simulink model "linear_Einspurmodel"  (R2025b)
settings: Solver=ode4  StartTime=0.0  StopTime=400  FixedStep=5e-05  RelTol=1e-8
values from neighbouring files (symbols this model uses):
  v = 18    [Aufgabe4.m]
settings Model: Creator=jonas  LastModifiedBy=fisch
settings DataIOCC: ExternalInput=u_ext  LoadExternalInput=on

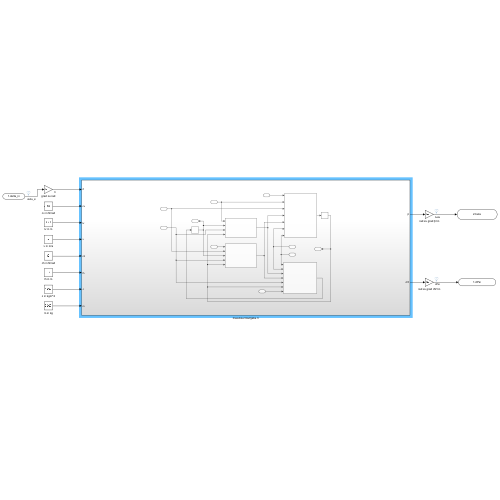
[thumbnail: Simulink's stored preview of the top-level diagram]
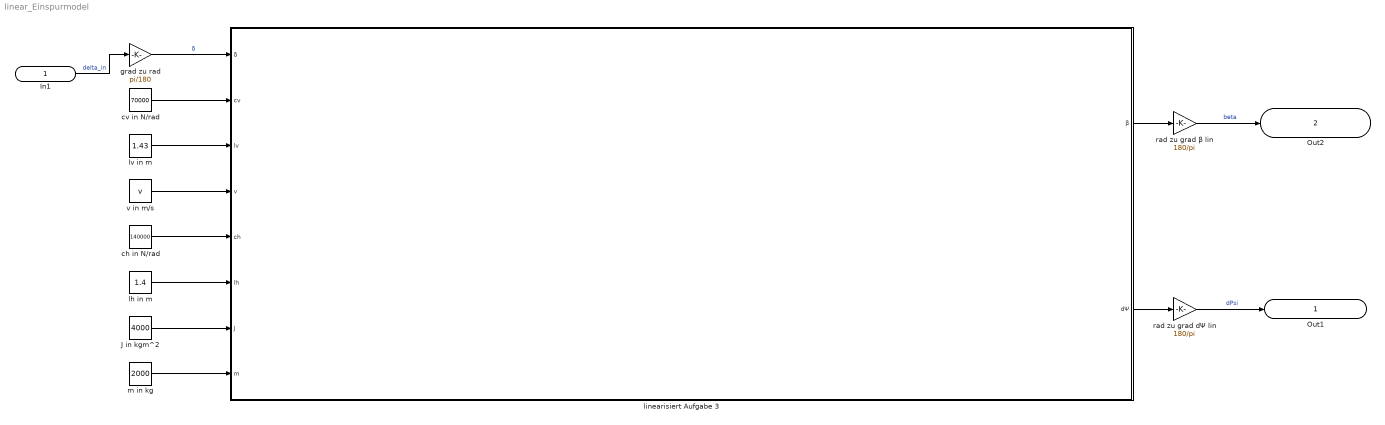
== system linear_Einspurmodel ==
  In1 : Inport
  J in kgm^2 : Constant  Value=4000
  ch in N/rad : Constant  Value=140000
  cv in N/rad : Constant  Value=70000
  grad zu rad : Gain  Gain=pi/180
  lh in m : Constant  Value=1.4
  linearisiert Aufgabe 3 : Subsystem
  lv in m : Constant  Value=1.43
  m in kg : Constant  Value=2000
  rad zu grad dΨ lin : Gain  Gain=180/pi
  rad zu grad β lin : Gain  Gain=180/pi
  v in m/s : Constant  Value=v
  Out1 : Outport
  Out2 : Outport  Port=2
  wires:
  In1/1 -> grad zu rad/1  "delta_in"
  grad zu rad/1 -> linearisiert Aufgabe 3/1(δ)  "δ"
  cv in N/rad/1 -> linearisiert Aufgabe 3/2(cv)
  lv in m/1 -> linearisiert Aufgabe 3/3(lv)
  v in m/s/1 -> linearisiert Aufgabe 3/4(v)
  ch in N/rad/1 -> linearisiert Aufgabe 3/5(ch)
  lh in m/1 -> linearisiert Aufgabe 3/6(lh)
  J in kgm^2/1 -> linearisiert Aufgabe 3/7(J)
  m in kg/1 -> linearisiert Aufgabe 3/8(m)
  linearisiert Aufgabe 3/1(β) -> rad zu grad β lin/1
  linearisiert Aufgabe 3/2(dΨ) -> rad zu grad dΨ lin/1
  rad zu grad dΨ lin/1 -> Out1/1  "dPsi"
  rad zu grad β lin/1 -> Out2/1  "beta"

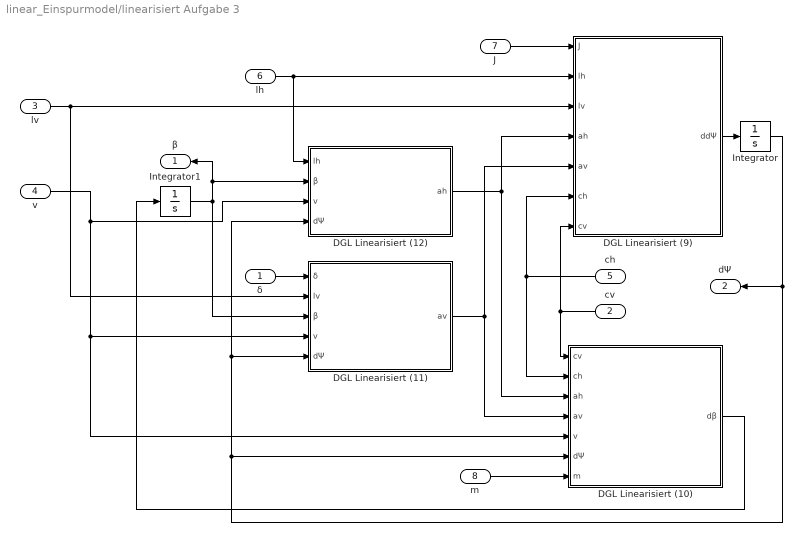
== system linear_Einspurmodel/linearisiert Aufgabe 3 ==
  δ : Inport
  cv : Inport  Port=2
  lv : Inport  Port=3
  v : Inport  Port=4
  ch : Inport  Port=5
  lh : Inport  Port=6
  J : Inport  Port=7
  m : Inport  Port=8
  DGL Linearisiert (10) : Subsystem
  DGL Linearisiert (11) : Subsystem
  DGL Linearisiert (12) : Subsystem
  DGL Linearisiert (9) : Subsystem
  Integrator : Integrator
  Integrator1 : Integrator
  β : Outport
  dΨ : Outport  Port=2
  wires:
  DGL Linearisiert (10)/1(dβ) -> Integrator1/1
  DGL Linearisiert (12)/1(ah) -> DGL Linearisiert (10)/3(ah), DGL Linearisiert (9)/4(ah)
  ch/1 -> DGL Linearisiert (9)/6(ch), DGL Linearisiert (10)/2(ch)
  Integrator/1 -> DGL Linearisiert (10)/6(dΨ), DGL Linearisiert (11)/5(dΨ), DGL Linearisiert (12)/4(dΨ), dΨ/1
  DGL Linearisiert (9)/1(ddΨ) -> Integrator/1
  Integrator1/1 -> DGL Linearisiert (12)/2(β), β/1, DGL Linearisiert (11)/3(β)
  δ/1 -> DGL Linearisiert (11)/1(δ)
  lh/1 -> DGL Linearisiert (12)/1(lh), DGL Linearisiert (9)/2(lh)
  DGL Linearisiert (11)/1(av) -> DGL Linearisiert (10)/4(av), DGL Linearisiert (9)/5(av)
  lv/1 -> DGL Linearisiert (11)/2(lv), DGL Linearisiert (9)/3(lv)
  cv/1 -> DGL Linearisiert (9)/7(cv), DGL Linearisiert (10)/1(cv)
  J/1 -> DGL Linearisiert (9)/1(J)
  v/1 -> DGL Linearisiert (10)/5(v), DGL Linearisiert (11)/4(v), DGL Linearisiert (12)/3(v)
  m/1 -> DGL Linearisiert (10)/7(m)

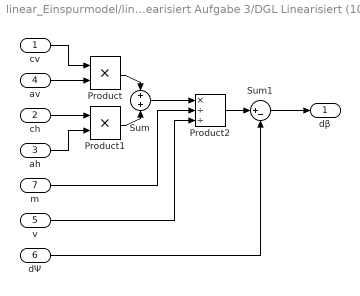
== system linear_Einspurmodel/linearisiert Aufgabe 3/DGL Linearisiert (10) ==
  cv : Inport
  ch : Inport  Port=2
  ah : Inport  Port=3
  av : Inport  Port=4
  v : Inport  Port=5
  dΨ : Inport  Port=6
  m : Inport  Port=7
  Product : Product  Inputs=**
  Product1 : Product  Inputs=**
  Product2 : Product  Inputs=*//
  Sum : Sum  Inputs=+|+
  Sum1 : Sum  Inputs=|+-
  dβ : Outport
  wires:
  Product/1 -> Sum/1
  m/1 -> Product2/2
  cv/1 -> Product/1
  Product2/1 -> Sum1/1
  Product1/1 -> Sum/2
  Sum/1 -> Product2/1
  Sum1/1 -> dβ/1
  av/1 -> Product/2
  v/1 -> Product2/3
  dΨ/1 -> Sum1/2
  ah/1 -> Product1/2
  ch/1 -> Product1/1

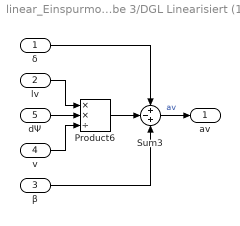
== system linear_Einspurmodel/linearisiert Aufgabe 3/DGL Linearisiert (11) ==
  δ : Inport
  lv : Inport  Port=2
  β : Inport  Port=3
  v : Inport  Port=4
  dΨ : Inport  Port=5
  Product6 : Product  Inputs=**/
  Sum3 : Sum  Inputs=+-+
  av : Outport
  wires:
  lv/1 -> Product6/1
  β/1 -> Sum3/3
  Product6/1 -> Sum3/2
  dΨ/1 -> Product6/2
  Sum3/1 -> av/1  "av"
  v/1 -> Product6/3
  δ/1 -> Sum3/1

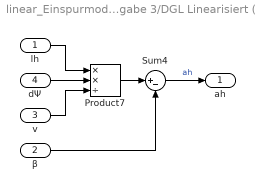
== system linear_Einspurmodel/linearisiert Aufgabe 3/DGL Linearisiert (12) ==
  lh : Inport
  β : Inport  Port=2
  v : Inport  Port=3
  dΨ : Inport  Port=4
  Product7 : Product  Inputs=**/
  Sum4 : Sum  Inputs=|+-
  ah : Outport
  wires:
  Product7/1 -> Sum4/1
  dΨ/1 -> Product7/2
  β/1 -> Sum4/2
  lh/1 -> Product7/1
  v/1 -> Product7/3
  Sum4/1 -> ah/1  "ah"

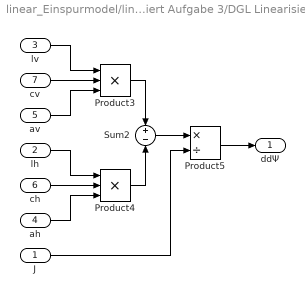
== system linear_Einspurmodel/linearisiert Aufgabe 3/DGL Linearisiert (9) ==
  J : Inport
  lh : Inport  Port=2
  lv : Inport  Port=3
  ah : Inport  Port=4
  av : Inport  Port=5
  ch : Inport  Port=6
  cv : Inport  Port=7
  Product3 : Product  Inputs=***
  Product4 : Product  Inputs=***
  Product5 : Product  Inputs=*/
  Sum2 : Sum  Inputs=+|-
  ddΨ : Outport
  wires:
  Sum2/1 -> Product5/1
  av/1 -> Product3/3
  ch/1 -> Product4/2
  lh/1 -> Product4/1
  Product3/1 -> Sum2/1
  cv/1 -> Product3/2
  Product4/1 -> Sum2/2
  ah/1 -> Product4/3
  Product5/1 -> ddΨ/1
  lv/1 -> Product3/1
  J/1 -> Product5/2
